simulink model "finalinversorPalacios"  (R2017a)
settings: Solver=ode3  StartTime=0.0  StopTime=10  MaxStep=1e-4  RelTol=1e-3
values from neighbouring files (symbols this model uses):
  Al = [0 -Uss/L; Uss/C -1/(R*C)]    [sistemacontrolado.m]    (also in sistemacontrolado.mat = [0  -0.441941738242; 441.941738242  -34.7222222222])
  Bl = [-X2ss/L; X1ss/C]    [sistemacontrolado.m]    (also in sistemacontrolado.mat = [-339.41125497 38.4])
  C = Ca1    (= 0.001)    [sistemacontrolado.m]    (also in sistemacontrolado.mat)
  C1 = 1.1e-6    (= 1.1e-06)    [sistemacontrolado.m]    (also in sistemacontrolado.mat)
  CI = x(end,1:2)    [sistemacontrolado.m]    (also in sistemacontrolado.mat = [0.0768083670357 339.401981032])
  Cl = [0 1]    [sistemacontrolado.m]    (also in sistemacontrolado.mat)
  I1 = 1.17    [sistemacontrolado.m]    (also in sistemacontrolado.mat)
  I2 = 3    [sistemacontrolado.m]    (also in sistemacontrolado.mat)
  Ki = k(1,3)    [sistemacontrolado.m]    (also in sistemacontrolado.mat = 8.5)
  Kp = k(1,1:2)    [sistemacontrolado.m]    (also in sistemacontrolado.mat = [-1.69344903458 -0.221299069674])
  L = 1    [sistemacontrolado.m]    (also in sistemacontrolado.mat)
  L1 = 4.5e-3    (= 0.0045)    [sistemacontrolado.m]    (also in sistemacontrolado.mat)
  La = 3e-3    (= 0.003)    [sistemacontrolado.m]    (also in sistemacontrolado.mat)
  R = Ra1    (= 28.8)    [sistemacontrolado.m]    (also in sistemacontrolado.mat)
  R1 = 1    [sistemacontrolado.m]    (also in sistemacontrolado.mat)
libraries: powerlib x56, fl_lib x5, nesl_utility x4, powerlib_extras x2, simulink x2, mpclib x1
settings Model: Creator=Administrador  LastModifiedBy=AndrewB
settings OptimizationCC: LifeSpan=inf
settings DebuggingCC: MaxConsecutiveZCsMsg=warning  SFExecutionAtInitializationDiag=none

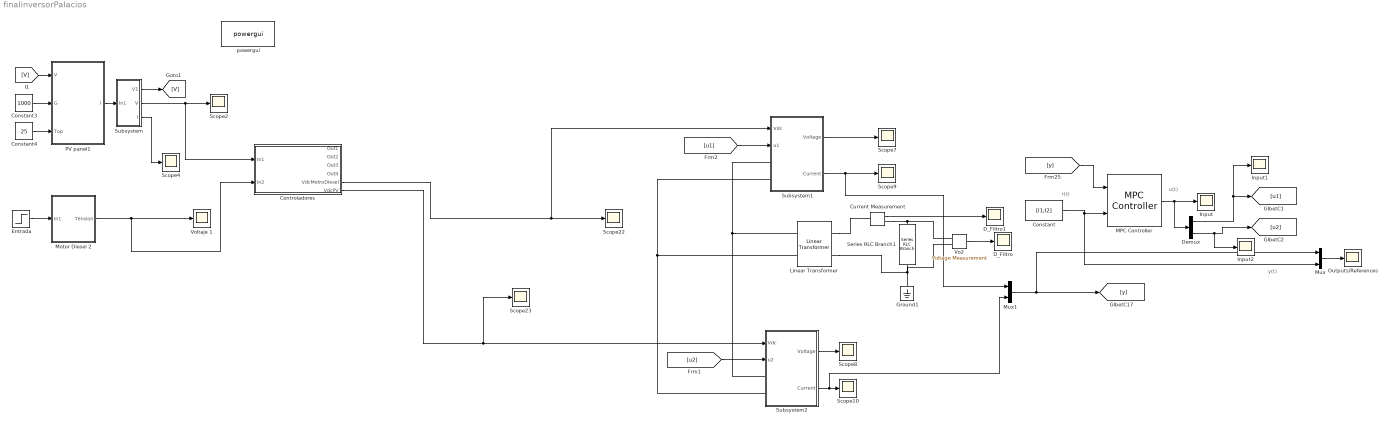
== system finalinversorPalacios ==
  note: u(t)
  note: y(t)
  note: r(t)
  Constant : Constant  Value=[I1;I2]
  Constant3 : Constant  Value=1000
  Constant4 : Constant  Value=25
  Controladores : Subsystem
  Current Measurement : powerlib/Measurements/Current Measurement  PhasorSimulation=off  OutputType=Complex  PSBequivalent=0
  D_Filtro : Scope
  D_Filtro1 : Scope
  Demux : Demux  Outputs=2
  Entrada : Step  Time=0  SampleTime=0
  Ground1 : powerlib/Elements/Ground  LConnTagsString=a
  Input : Scope
  Input1 : Scope
  Input2 : Scope
  Linear Transformer : powerlib/Elements/Linear Transformer  UNITS=SI  NominalPower=[ 1500 60 ]  winding1=[141.2 0 0.003]  winding2=[120 0.004 0.084225]  ThreeWindings=off  winding3=[3.15e+05 0.7938 0.084225]  RmLm=[1.0805e+06 2866]  Measurements=None  DataType=on
  MPC Controller : mpclib/MPC Controller  mpcobj=mpcobj  x0=[]  is_multiple=0  enable_value=0  return_u0=off  ref_from_ws=off  ref_signal_name=[]  ref_preview=on  md_from_ws=off  md_signal_name=[]  md_preview=on  from_project=off  project_file=MPCtask.mat  md_inport=off  mv_inport=off  cost_outport=off  return_sequence=off  return_qpstatus=off  return_state=off  state_inport=off  lims_inport=off  ywt_inport=off  is_designfromscratch=0  uwt_inport=off  duwt_inport=off  rhoeps_inport=off  uref_inport=off  n_ts=0.1  n_mv=2  n_md=0  n_ud=0  n_mo=2  n_uo=0  BlockDataType=double  SampleTimeInherited=off  switch_inport=off
  Motor Diesel 2 : Subsystem
  Mux : Mux  Inputs=2
  Mux1 : Mux  Inputs=2
  Outputs/References : Scope
  PV panel1 : Subsystem
      mask Display: image('panel.jpg')
  Scope{2,4,7..10,22..23} (8 alike) : Scope
  Series RLC Branch1 : powerlib/Elements/Series RLC Branch  LConnTagsString=__new0  RConnTagsString=__new0  BranchType=R  Resistance=R  Inductance=25e-3  SetiL0=off  InitialCurrent=0  Capacitance=5.30e-3  Setx0=off  InitialVoltage=0  Measurements=None
  Subsystem : Subsystem
  Subsystem1 : Subsystem
  Subsystem2 : Subsystem
  Vo2 : powerlib/Measurements/Voltage Measurement  PhasorSimulation=off  OutputType=Complex  PSBequivalent=0
  Voltaje 1 : Scope
  powergui : powerlib/powergui  SimulationMode=Discrete  SampleTime=1/60/10000  frequency=60  Iterations=50  frequencyindice=0  Pbase=100e6  ErrMax=1e-4  UnitsV=kV  UnitsW=MW  buscounter=0  FunctionMessages=off  echomessages=off  EnableUseOfTLC=off  CurrentSourceSwitches=off  DisableSnubberDevices=off  DisableRonSwitches=off  DisableVfSwitches=off  DisplayEquations=off  SolverType=Tustin/Backward Euler (TBE)  Interpol=off  ExternalGateDelay=off  methode=off  Ts=100  x0status=blocks  SPID=on  SwTol=0  HookPort=off  RestoreLinks=warning  ResistiveCurrentMeasurement=off  Frange=[0:2:500]  Ylog=off  Xlog=on  ShowGrid=off  save=off  variable=ZData  structure=sps1phPWM1_str  ZoomFFT=on  StartTime=0.1-2/60  cycles=2  DisplayStyle=1  fundamental=60  FreqAxis=off  MaxFrequency=5000  frequencyindicesteady=1  RmsSteady=1  display=off
  wires:
  [V] -> PV panel1/1(V)
  Subsystem/1(V1) -> [V]
  Constant4/1 -> PV panel1/3(Top)
  PV panel1/1(I) -> Subsystem/1(In1)
  Constant3/1 -> PV panel1/2(G)
  Subsystem/2(V) -> Controladores/1(In1), Scope2/1
  Subsystem/3(I) -> Scope4/1
  Entrada/1 -> Motor Diesel 2/1(In1)
  Motor Diesel 2/1(Tension) -> Controladores/2(In2), Voltaje 1/1
  Subsystem1/1(Voltage) -> Scope7/1
  Subsystem1/2(Current) -> Mux1/1, Scope9/1
  Vo2/1 -> D_Filtro/1
  Subsystem2/1(Voltage) -> Scope8/1
  Subsystem2/2(Current) -> Mux1/2, Scope10/1
  Current Measurement/1 -> D_Filtro1/1
  MPC Controller/1 -> Demux/1, Input/1
  Constant/1 -> Mux/2, MPC Controller/2
  Mux/1 -> Outputs/References/1
  [y] -> MPC Controller/1
  Mux1/1 -> Mux/1, [y]
  Demux/1 -> Input1/1, [u1]
  Demux/2 -> Input2/1, [u2]
  [u2] -> Subsystem2/2("u2 ")
  [u1] -> Subsystem1/2(u1)
  Controladores/5(VdcMotroDiesel) -> Subsystem1/1(Vdc), Scope22/1
  Controladores/6(VdcPV) -> Subsystem2/1(Vdc), Scope23/1
  connections:
  Subsystem1/LConn1 -- Subsystem2/LConn1 -- Linear Transformer/LConn1
  Subsystem1/LConn2 -- Subsystem2/LConn2 -- Linear Transformer/LConn2
  Vo2/LConn1 -- Current Measurement/RConn1 -- Series RLC Branch1/LConn1
  Ground1/LConn1 -- Linear Transformer/RConn2 -- Vo2/LConn2 -- Series RLC Branch1/RConn1
  Linear Transformer/RConn1 -- Current Measurement/LConn1

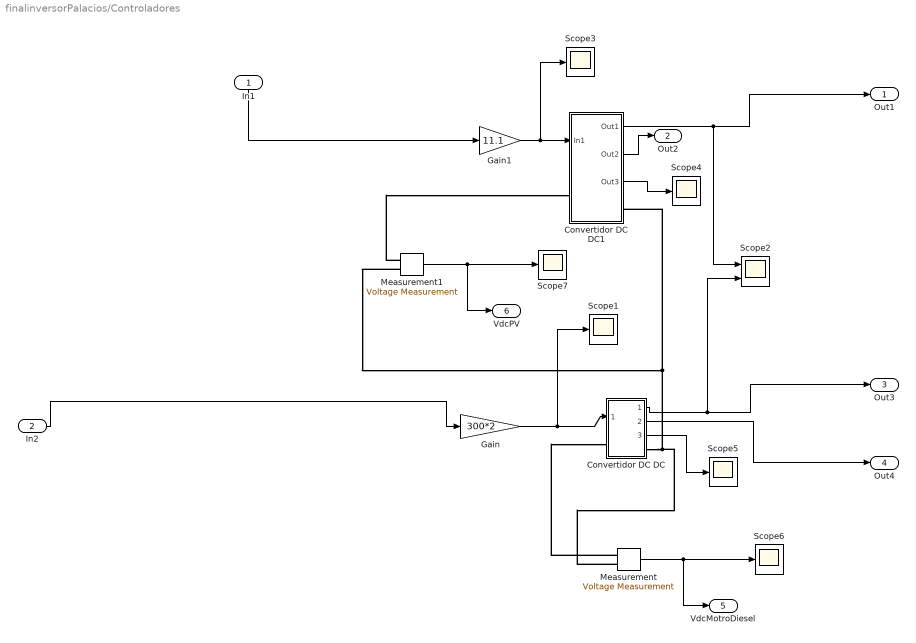
== system finalinversorPalacios/Controladores ==
  In1 : Inport
  In2 : Inport  Port=2
  " Measurement" : powerlib/Measurements/Voltage Measurement  PhasorSimulation=off  OutputType=Complex  PSBequivalent=0
  " Measurement1" : powerlib/Measurements/Voltage Measurement  PhasorSimulation=off  OutputType=Complex  PSBequivalent=0
  Convertidor DC DC : Subsystem
  Convertidor DC DC1 : Subsystem
  Gain : Gain  Gain=300*2
  Gain1 : Gain  Gain=11.1
  Scope{1,3..7} (6 alike) : Scope
  Scope2 : Scope  NumInputPorts=2
  Out1 : Outport
  Out2 : Outport  Port=2
  Out3 : Outport  Port=3
  Out4 : Outport  Port=4
  VdcMotroDiesel : Outport  Port=5
  VdcPV : Outport  Port=6
  wires:
  Gain/1 -> Scope1/1, Convertidor DC DC/1(In1)
  Convertidor DC DC/1(Out1) -> Scope2/2, Out3/1
  Convertidor DC DC1/1(Out1) -> Out1/1, Scope2/1
  Gain1/1 -> Scope3/1, Convertidor DC DC1/1(In1)
  Convertidor DC DC/2(Out2) -> Out4/1
  Convertidor DC DC1/2(Out2) -> Out2/1
  In1/1 -> Gain1/1
  In2/1 -> Gain/1
  Convertidor DC DC1/3(Out3) -> Scope4/1
  Convertidor DC DC/3(Out3) -> Scope5/1
  " Measurement"/1 -> VdcMotroDiesel/1, Scope6/1
  " Measurement1"/1 -> VdcPV/1, Scope7/1
  connections:
  Convertidor DC DC/RConn1 -- " Measurement"/LConn2 -- " Measurement1"/LConn2 -- Convertidor DC DC1/RConn1
  " Measurement"/LConn1 -- Convertidor DC DC/LConn1
  " Measurement1"/LConn1 -- Convertidor DC DC1/LConn1

== system finalinversorPalacios/Motor Diesel 2 ==
  In1 : Inport
  " Generador1" : Gain  Gain=1/2
  Actuador1 : TransferFcn  Denominator=[0.2 1]
  Control PI : TransferFcn  Numerator=[1 0.653]  Denominator=[1 0]
  Gain : Gain  Gain=3.87
  Inercia y fricción1 : TransferFcn  Denominator=[2.5 0.1]
  Scope1 : Scope
  Scope2 : Scope
  Scope3 : Scope
  Sistema de combustión1 : TransportDelay  DelayTime=0.1
  Sum : Sum  Inputs=|+-
  Tension : Outport
  wires:
  " Generador1"/1 -> Tension/1
  Actuador1/1 -> Sistema de combustión1/1, Scope2/1
  Gain/1 -> Control PI/1
  Sum/1 -> Gain/1
  Inercia y fricción1/1 -> Scope3/1, " Generador1"/1, Sum/2
  Control PI/1 -> Actuador1/1
  In1/1 -> Sum/1
  Sistema de combustión1/1 -> Inercia y fricción1/1, Scope1/1

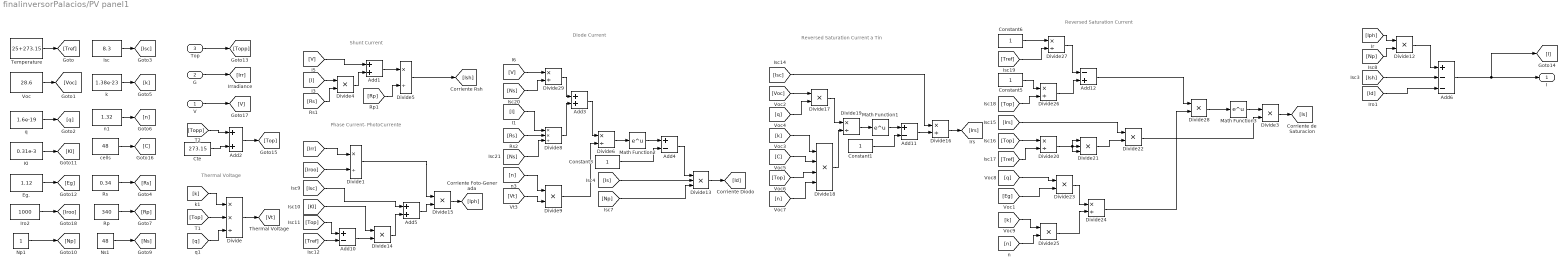
== system finalinversorPalacios/PV panel1 ==
  note: Thermal Voltage
  note: Shunt Current
  note: Phase Current- PhotoCurrente
  note: Diode Current
  note: Reversed Saturation Current a Tin
  note: Reversed Saturation Current
  V : Inport
  G : Inport  Port=2
  Top : Inport  Port=3
  Add{1..3,5} (4 alike) : Sum
  Add10 : Sum  Inputs=+-
  Add11 : Sum  Inputs=+-
  Add12 : Sum  Inputs=-+
  Add4 : Sum  Inputs=+-
  Add6 : Sum  Inputs=+--
  Constant{1,3,5..6} (4 alike) : Constant
  Cte : Constant  Value=273.15
  Divide : Product  Inputs=**/
  Divide{1,5..6,16,19..20,24,26..27,29} (10 alike) : Product  Inputs=*/
  Divide{3..4,9,12,14..15,17,22..23,25,28} (11 alike) : Product  Inputs=**
  Divide13 : Product  Inputs=***
  Divide18 : Product  Inputs=****
  Divide21 : Product  Inputs=***
  Divide8 : Product  Inputs=**/
  Eg. : Constant  Value=1.12
  Iro2 : Constant  Value=1000
  Isc : Constant  Value=8.3
  KI : Constant  Value=0.31e-3
  Math Function1 : Math  SaturateOnIntegerOverflow=on
  Math Function2 : Math  SaturateOnIntegerOverflow=on
  Math Function3 : Math  SaturateOnIntegerOverflow=on
  Np1 : Constant
  Ns1 : Constant  Value=48
  Rp : Constant  Value=340
  Rs : Constant  Value=0.34
  Temperature : Constant  Value=25+273.15
  Voc : Constant  Value=28.6
  cells : Constant  Value=48
  k : Constant  Value=1.38e-23
  n1 : Constant  Value=1.32
  q : Constant  Value=1.6e-19
  I : Outport
  wires:
  Temperature/1 -> [Tref]
  Voc/1 -> [Voc]
  q/1 -> [q]
  Isc/1 -> [Isc]
  k/1 -> [k]
  n1/1 -> [n]
  [k] -> Divide/1
  [Top] -> Divide/2
  [q] -> Divide/3
  Divide/1 -> [Vt]
  Divide3/1 -> [Is]
  [Ish] -> Add6/2
  Add6/1 -> I/1, [I]
  [I] -> Divide8/1
  [Rs] -> Divide8/2
  Divide8/1 -> Add3/2
  [n] -> Divide9/1
  [Vt] -> Divide9/2
  Divide9/1 -> Divide6/2
  Add3/1 -> Divide6/1
  Divide6/1 -> Math Function2/1
  Math Function2/1 -> Add4/1
  Add4/1 -> Divide13/1
  [Is] -> Divide13/2
  Divide13/1 -> [Id]
  Divide4/1 -> Add1/2
  Add1/1 -> Divide5/1
  [Rp] -> Divide5/2
  Divide5/1 -> [Ish]
  [Rs] -> Divide4/2
  [I] -> Divide4/1
  KI/1 -> [KI]
  Eg./1 -> [Eg]
  [V] -> Add1/1
  [Np] -> Divide13/3
  [Iph] -> Divide12/1
  [Np] -> Divide12/2
  Divide12/1 -> Add6/1
  [Isc] -> Add5/1
  [Top] -> Add10/1
  [Tref] -> Add10/2
  Add10/1 -> Divide14/2
  [KI] -> Divide14/1
  [Voc] -> Divide17/1
  [q] -> Divide17/2
  [k] -> Divide18/1
  [C] -> Divide18/2
  [Top] -> Divide18/3
  [n] -> Divide18/4
  Divide17/1 -> Divide19/1
  Divide18/1 -> Divide19/2
  Divide19/1 -> Math Function1/1
  Constant1/1 -> Add11/2
  Math Function1/1 -> Add11/1
  Add11/1 -> Divide16/2
  Divide16/1 -> [Irs]
  [Tref] -> Divide20/2
  [Top] -> Divide20/1
  Divide20/1 -> Divide21/2, Divide21/1, Divide21/3
  Divide21/1 -> Divide22/2
  [Irs] -> Divide22/1
  [q] -> Divide23/1
  Divide23/1 -> Divide24/1
  [k] -> Divide25/1
  [n] -> Divide25/2
  Divide25/1 -> Divide24/2
  Constant5/1 -> Divide26/1
  [Top] -> Divide26/2
  Constant6/1 -> Divide27/1
  [Tref] -> Divide27/2
  Divide27/1 -> Add12/1
  Divide26/1 -> Add12/2
  Add12/1 -> Divide28/1
  Divide24/1 -> Divide28/2
  Divide28/1 -> Math Function3/1
  Divide29/1 -> Add3/1
  [Ns] -> Divide29/2
  [V] -> Divide29/1
  [Ns] -> Divide8/3
  Divide14/1 -> Add5/2
  Add5/1 -> Divide15/2
  Divide15/1 -> [Iph]
  V/1 -> [V]
  G/1 -> [Irr]
  Top/1 -> [Topp]
  cells/1 -> [C]
  [Id] -> Add6/3
  Cte/1 -> Add2/2
  Add2/1 -> [Top]
  [Topp] -> Add2/1
  [Irr] -> Divide1/1
  [Iroo] -> Divide1/2
  Divide1/1 -> Divide15/1
  Iro2/1 -> [Iroo]
  Rs/1 -> [Rs]
  Rp/1 -> [Rp]
  Ns1/1 -> [Ns]
  Np1/1 -> [Np]
  Constant3/1 -> Add4/2
  [Isc] -> Divide16/1
  Math Function3/1 -> Divide3/1
  Divide22/1 -> Divide3/2
  [Eg] -> Divide23/2

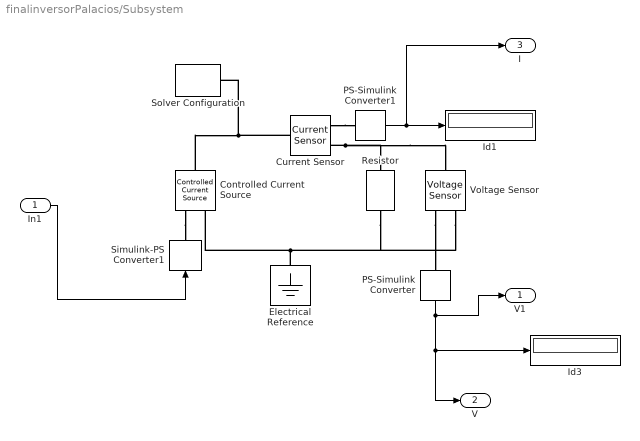
== system finalinversorPalacios/Subsystem ==
  In1 : Inport
  Controlled Current Source : fl_lib/Electrical/Electrical Sources/Controlled Current Source
  Current Sensor : fl_lib/Electrical/Electrical Sensors/Current Sensor
  Electrical Reference : fl_lib/Electrical/Electrical Elements/Electrical Reference
  Id1 : Display
  Id3 : Display
  PS-Simulink Converter : nesl_utility/PS-Simulink Converter  PhysicalDomain=network_engine_domain  SubClassName=ps_output  LeftPortType=input  RightPortType=output  PseudoPeriodic=off  Frequencies=[]  Unit=1  AffineConversion=off
  PS-Simulink Converter1 : nesl_utility/PS-Simulink Converter  PhysicalDomain=network_engine_domain  SubClassName=ps_output  LeftPortType=input  RightPortType=output  PseudoPeriodic=off  Frequencies=[]  Unit=1  AffineConversion=off
  Resistor : fl_lib/Electrical/Electrical Elements/Resistor  R=10.02 Ohm  i_specify=off  i_priority=High  i=0 A  i_nominal_specify=off  i_nominal_unit=A  i_nominal_value=1  v_specify=off  v_priority=High  v=0 V  v_nominal_specify=off  v_nominal_unit=V  v_nominal_value=1
  Simulink-PS Converter1 : nesl_utility/Simulink-PS Converter  PhysicalDomain=network_engine_domain  SubClassName=ps_input  LeftPortType=input  RightPortType=output  PseudoPeriodic=off  Frequencies=[]  NoiseDistribution=none  NoiseParameters=[]  Unit=1  AffineConversion=off  FilteringAndDerivatives=zero  SimscapeFilterOrder=1  InputFilterTimeConstant=.000001  UdotUserProvided=0
  Solver Configuration : nesl_utility/Solver Configuration  PhysicalDomain=network_engine_domain  SubClassName=solver  LeftPortType=input  RightPortType=generic  Accelerate=off  Tones=[]  Harmonics=[]  SimulateNoise=off  Profile=off  UseLocalSampling=off  EnableSwitchedLinearOptims=on  FrequencyDomain=off  UseCCode=off  RelTol=0.001  AbsTol=1e-06  MinStep=1e-09  ToWorkspace=off  RevertToSquareIcSolve=off  NumHomotopyIterations=100  PhasorMode=off  PhasorModeNumHarmonics=1  OverrideAbsTol=off  DoDC=on  ResidualTolerance=1e-8  UseLocalSolver=on  LocalSolverChoice=NE_BACKWARD_EULER_ADVANCER  LocalSolverSampleTime=.1  DoFixedCost=off  MaxNonlinIter=8  MaxModeIter=2  LinearAlgebra=Sparse  DelaysMemoryBudget=1024  AutomaticFiltering=on  FilteringTimeConstant=0.001
  Voltage Sensor : fl_lib/Electrical/Electrical Sensors/Voltage Sensor
  V1 : Outport
  V : Outport  Port=2
  I : Outport  Port=3
  wires:
  PS-Simulink Converter1/1 -> I/1, Id1/1
  PS-Simulink Converter/1 -> V1/1, V/1, Id3/1
  In1/1 -> Simulink-PS Converter1/1
  connections:
  Voltage Sensor/RConn1 -- PS-Simulink Converter/LConn1
  Current Sensor/RConn2 -- Voltage Sensor/LConn1 -- Resistor/LConn1
  Controlled Current Source/RConn1 -- Simulink-PS Converter1/RConn1
  Electrical Reference/LConn1 -- Voltage Sensor/RConn2 -- Resistor/RConn1 -- Controlled Current Source/RConn2
  Current Sensor/RConn1 -- PS-Simulink Converter1/LConn1
  Controlled Current Source/LConn1 -- Current Sensor/LConn1 -- Solver Configuration/RConn1

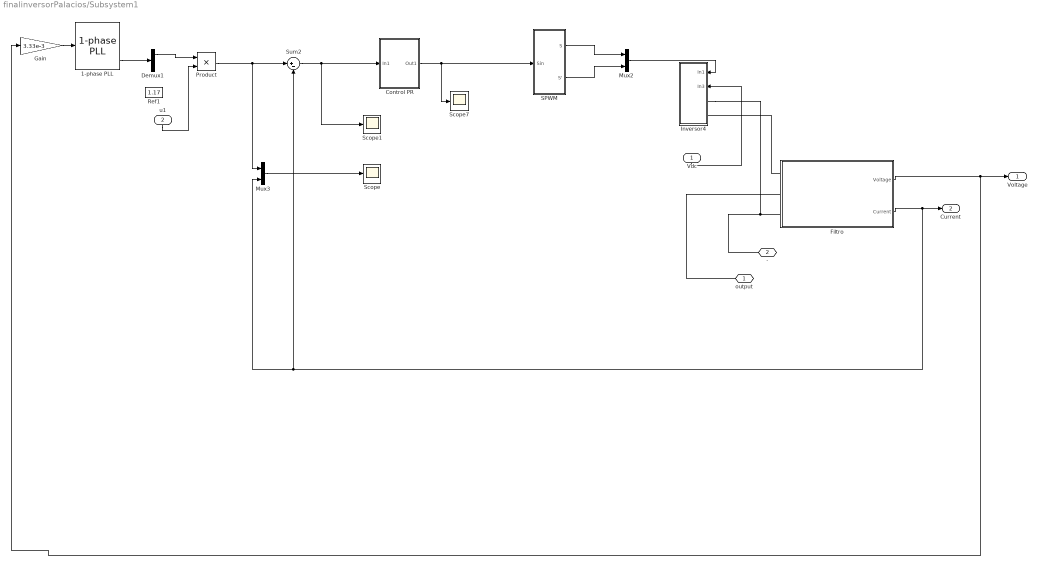
== system finalinversorPalacios/Subsystem1 ==
  Vdc : Inport
  u1 : Inport  Port=2
  1-phase PLL : powerlib_extras/Control  Blocks/1-phase PLL  Par_Init=[0 60]  ParK=[ 180 3200 1 ]  AGC=off
  Control PR : Subsystem
  Demux1 : Demux  Outputs=2
  Filtro : Subsystem
  Gain : Gain  Gain=3.33e-3
  Inversor4 : Subsystem
  Mux2 : Mux  Inputs=2
  Mux3 : Mux  Inputs=2
  Product : Product
  Ref1 : Constant  Value=1.17
  SPWM : Subsystem
  Scope : Scope
  Scope1 : Scope
  Scope7 : Scope
  Sum2 : Sum  Inputs=|+-
  output : PMIOPort  Port=1  Side=Left
  - : PMIOPort  Port=2  Side=Left
  Voltage : Outport
  Current : Outport  Port=2
  wires:
  Filtro/2(Current) -> Mux3/2, Sum2/2, Current/1
  Filtro/1(Voltage) -> Gain/1, Voltage/1
  1-phase PLL/3 -> Demux1/1
  Gain/1 -> 1-phase PLL/1
  Mux3/1 -> Scope/1
  Product/1 -> Mux3/1, Sum2/1
  Demux1/1 -> Product/1
  SPWM/1(S) -> Mux2/1
  SPWM/2(S') -> Mux2/2
  Mux2/1 -> Inversor4/1(In1)
  Vdc/1 -> Inversor4/2(In3)
  Control PR/1(Out1) -> Scope7/1, SPWM/1(Sin)
  Sum2/1 -> Scope1/1, Control PR/1(In1)
  u1/1 -> Product/2
  connections:
  output/RConn1 -- Filtro/LConn2
  -/RConn1 -- Inversor4/LConn1 -- Filtro/LConn3
  Filtro/LConn1 -- Inversor4/LConn2

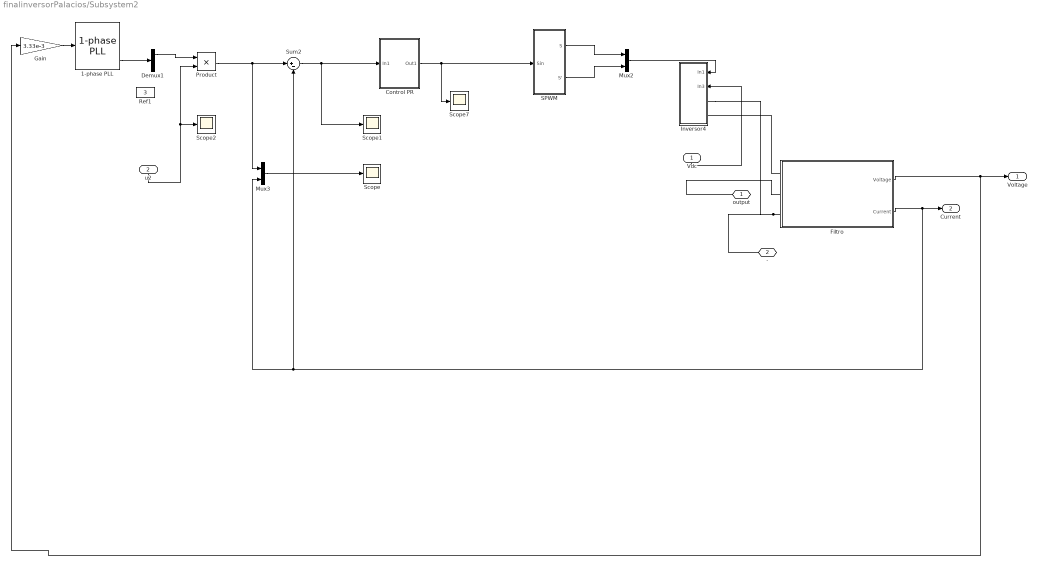
== system finalinversorPalacios/Subsystem2 ==
  Vdc : Inport
  "u2 " : Inport  Port=2
  1-phase PLL : powerlib_extras/Control  Blocks/1-phase PLL  Par_Init=[0 60]  ParK=[ 180 3200 1 ]  AGC=off
  Control PR : Subsystem
  Demux1 : Demux  Outputs=2
  Filtro : Subsystem
  Gain : Gain  Gain=3.33e-3
  Inversor4 : Subsystem
  Mux2 : Mux  Inputs=2
  Mux3 : Mux  Inputs=2
  Product : Product
  Ref1 : Constant  Value=3
  SPWM : Subsystem
  Scope{,1..2,7} (4 alike) : Scope
  Sum2 : Sum  Inputs=|+-
  output : PMIOPort  Port=1  Side=Left
  - : PMIOPort  Port=2  Side=Left
  Voltage : Outport
  Current : Outport  Port=2
  wires:
  Filtro/2(Current) -> Mux3/2, Sum2/2, Current/1
  Filtro/1(Voltage) -> Gain/1, Voltage/1
  1-phase PLL/3 -> Demux1/1
  Gain/1 -> 1-phase PLL/1
  Mux3/1 -> Scope/1
  Product/1 -> Mux3/1, Sum2/1
  Demux1/1 -> Product/1
  SPWM/1(S) -> Mux2/1
  SPWM/2(S') -> Mux2/2
  Mux2/1 -> Inversor4/1(In1)
  Vdc/1 -> Inversor4/2(In3)
  Control PR/1(Out1) -> Scope7/1, SPWM/1(Sin)
  Sum2/1 -> Scope1/1, Control PR/1(In1)
  "u2 "/1 -> Scope2/1, Product/2
  connections:
  output/RConn1 -- Filtro/LConn2
  Filtro/LConn3 -- -/RConn1 -- Inversor4/LConn1
  Filtro/LConn1 -- Inversor4/LConn2

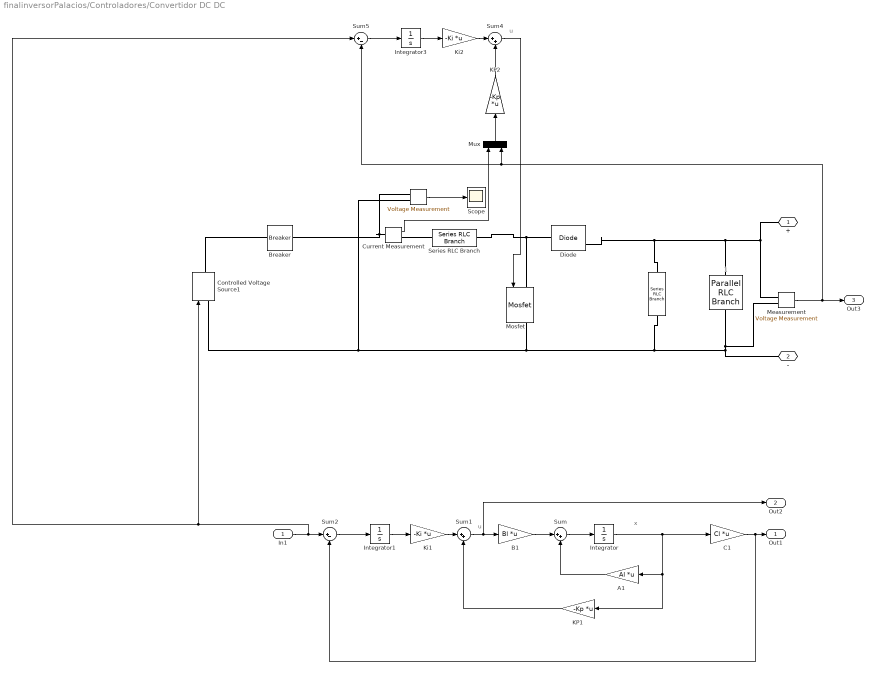
== system finalinversorPalacios/Controladores/Convertidor DC DC ==
  note: x
  note: u
  note: u
  In1 : Inport
  "  " : powerlib/Measurements/Voltage Measurement  PhasorSimulation=off  OutputType=Complex  PSBequivalent=0
  "    " : powerlib/Elements/Series RLC Branch  LConnTagsString=__new0  RConnTagsString=__new0  BranchType=C  Resistance=0  Inductance=69e-3  SetiL0=off  InitialCurrent=0  Capacitance=C  Setx0=off  InitialVoltage=0  Measurements=None
  "  1" : powerlib/Elements/Parallel RLC Branch  LConnTagsString=a  RConnTagsString=__new0  BranchType=R  Resistance=R  Inductance=1e-3  SetiL0=off  InitialCurrent=0  Capacitance=1e-6  Setx0=off  InitialVoltage=0  Measurements=None
  " Measurement" : powerlib/Measurements/Voltage Measurement  PhasorSimulation=off  OutputType=Complex  PSBequivalent=0
  A1 : Gain  Gain=Al  Multiplication=Matrix(K*u)
  B1 : Gain  Gain=Bl  Multiplication=Matrix(K*u)
  Breaker : powerlib/Elements/Breaker  InitialState=0  SwitchingTimes=[0 0.001]  External=off  BreakerResistance=0.01  SnubberResistance=1e6  SnubberCapacitance=inf  Measurements=None  MoreParameters=on  NoBreakLoop=off
      settings: SourceProductName=Simscape Power Systems
  C1 : Gain  Gain=Cl  Multiplication=Matrix(K*u)
  Controlled Voltage Source1 : powerlib/Electrical Sources/Controlled Voltage Source  Initialize=on  Source_Type=DC  Amplitude=0  Phase=0  Frequency=0  Measurements=None
  Current Measurement : powerlib/Measurements/Current Measurement  PhasorSimulation=off  OutputType=Complex  PSBequivalent=0
  Diode : powerlib/Power Electronics/Diode  Ron=0.001  Lon=0  Vf=0.8  IC=0  UseSnubber=off  Rs=500  Cs=250e-9  Measurements=on
  Integrator : Integrator  InitialCondition=CI
  Integrator1 : Integrator
  Integrator3 : Integrator
  KP1 : Gain  Gain=-Kp  Multiplication=Matrix(K*u)
  KP2 : Gain  Gain=-Kp  Multiplication=Matrix(K*u)
  Ki1 : Gain  Gain=-Ki  Multiplication=Matrix(K*u)
  Ki2 : Gain  Gain=-Ki  Multiplication=Matrix(K*u)
  Mosfet : powerlib/Power Electronics/Mosfet  Ron=0.1  Lon=0  Rd=0.01  Vfd=0  IC=0  Rs=1e5  Cs=inf  Measurements=on
  Mux : Mux  Inputs=2
  Scope : Scope
  Series RLC Branch : powerlib/Elements/Series RLC Branch  LConnTagsString=__new0  RConnTagsString=__new0  BranchType=L  Resistance=0  Inductance=L  SetiL0=off  InitialCurrent=0  Capacitance=1e-6  Setx0=off  InitialVoltage=0  Measurements=None
  Sum : Sum  Inputs=|++
  Sum1 : Sum  Inputs=|++
  Sum2 : Sum  Inputs=|+-
  Sum4 : Sum  Inputs=|++
  Sum5 : Sum  Inputs=|+-
  + : PMIOPort  Port=1  Side=Left
  - : PMIOPort  Port=2  Side=Right
  Out1 : Outport
  Out2 : Outport  Port=2
  Out3 : Outport  Port=3
  wires:
  Integrator1/1 -> Ki1/1
  B1/1 -> Sum/1
  Integrator/1 -> C1/1, KP1/1, A1/1
  Sum2/1 -> Integrator1/1
  Ki1/1 -> Sum1/1
  A1/1 -> Sum/2
  Sum/1 -> Integrator/1
  KP1/1 -> Sum1/2
  C1/1 -> Sum2/2, Out1/1
  Sum1/1 -> Out2/1, B1/1
  " Measurement"/1 -> Sum5/2, Mux/2, Out3/1
  In1/1 -> Sum5/1, Controlled Voltage Source1/1, Sum2/1
  "  "/1 -> Scope/1
  Mux/1 -> KP2/1
  Sum5/1 -> Integrator3/1
  Integrator3/1 -> Ki2/1
  Ki2/1 -> Sum4/1
  KP2/1 -> Sum4/2
  Sum4/1 -> Mosfet/1
  Current Measurement/1 -> Mux/1
  connections:
  Mosfet/RConn1 -- Controlled Voltage Source1/LConn1 -- "  "/LConn2 -- "    "/RConn1 -- -/RConn1 -- " Measurement"/LConn2 -- "  1"/RConn1
  "  1"/LConn1 -- +/RConn1 -- " Measurement"/LConn1 -- "    "/LConn1 -- Diode/RConn1
  Controlled Voltage Source1/RConn1 -- Breaker/LConn1
  Diode/LConn1 -- Series RLC Branch/RConn1 -- Mosfet/LConn1
  Current Measurement/RConn1 -- Series RLC Branch/LConn1
  Breaker/RConn1 -- Current Measurement/LConn1 -- "  "/LConn1

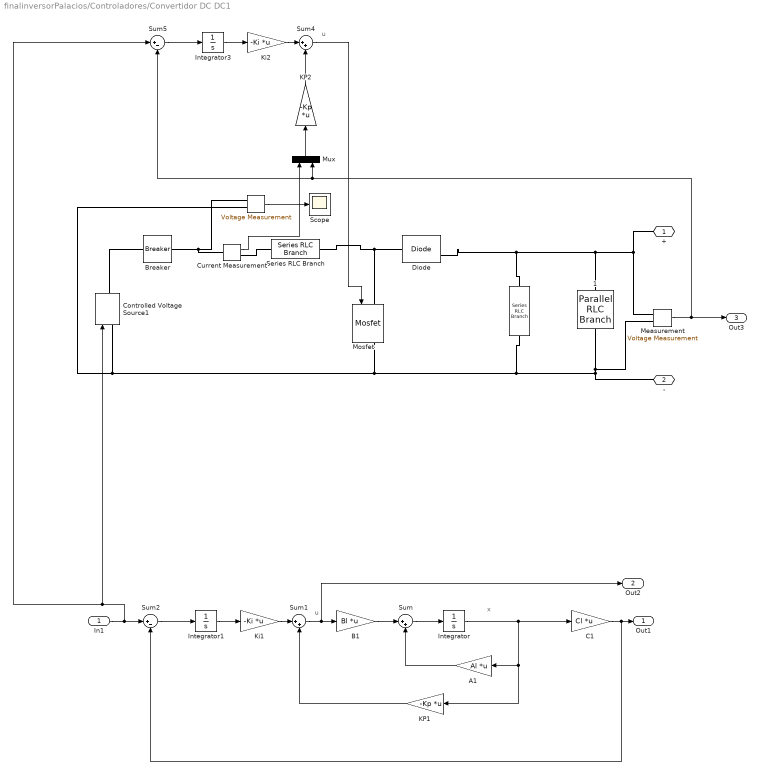
== system finalinversorPalacios/Controladores/Convertidor DC DC1 ==
  note: x
  note: u
  note: u
  In1 : Inport
  "  " : powerlib/Measurements/Voltage Measurement  PhasorSimulation=off  OutputType=Complex  PSBequivalent=0
  "    " : powerlib/Elements/Series RLC Branch  LConnTagsString=__new0  RConnTagsString=__new0  BranchType=C  Resistance=0  Inductance=69e-3  SetiL0=off  InitialCurrent=0  Capacitance=C  Setx0=off  InitialVoltage=0  Measurements=None
  "  1" : powerlib/Elements/Parallel RLC Branch  LConnTagsString=a  RConnTagsString=__new0  BranchType=R  Resistance=R  Inductance=1e-3  SetiL0=off  InitialCurrent=0  Capacitance=1e-6  Setx0=off  InitialVoltage=0  Measurements=None
  " Measurement" : powerlib/Measurements/Voltage Measurement  PhasorSimulation=off  OutputType=Complex  PSBequivalent=0
  A1 : Gain  Gain=Al  Multiplication=Matrix(K*u)
  B1 : Gain  Gain=Bl  Multiplication=Matrix(K*u)
  Breaker : powerlib/Elements/Breaker  InitialState=0  SwitchingTimes=[0 0.001]  External=off  BreakerResistance=0.01  SnubberResistance=1e6  SnubberCapacitance=inf  Measurements=None  MoreParameters=on  NoBreakLoop=off
      settings: SourceProductName=Simscape Power Systems
  C1 : Gain  Gain=Cl  Multiplication=Matrix(K*u)
  Controlled Voltage Source1 : powerlib/Electrical Sources/Controlled Voltage Source  Initialize=on  Source_Type=DC  Amplitude=0  Phase=0  Frequency=0  Measurements=None
  Current Measurement : powerlib/Measurements/Current Measurement  PhasorSimulation=off  OutputType=Complex  PSBequivalent=0
  Diode : powerlib/Power Electronics/Diode  Ron=0.001  Lon=0  Vf=0.8  IC=0  UseSnubber=off  Rs=500  Cs=250e-9  Measurements=on
  Integrator : Integrator  InitialCondition=CI
  Integrator1 : Integrator
  Integrator3 : Integrator
  KP1 : Gain  Gain=-Kp  Multiplication=Matrix(K*u)
  KP2 : Gain  Gain=-Kp  Multiplication=Matrix(K*u)
  Ki1 : Gain  Gain=-Ki  Multiplication=Matrix(K*u)
  Ki2 : Gain  Gain=-Ki  Multiplication=Matrix(K*u)
  Mosfet : powerlib/Power Electronics/Mosfet  Ron=0.1  Lon=0  Rd=0.01  Vfd=0  IC=0  Rs=1e5  Cs=inf  Measurements=on
  Mux : Mux  Inputs=2
  Scope : Scope
  Series RLC Branch : powerlib/Elements/Series RLC Branch  LConnTagsString=__new0  RConnTagsString=__new0  BranchType=L  Resistance=0  Inductance=L  SetiL0=off  InitialCurrent=0  Capacitance=1e-6  Setx0=off  InitialVoltage=0  Measurements=None
  Sum : Sum  Inputs=|++
  Sum1 : Sum  Inputs=|++
  Sum2 : Sum  Inputs=|+-
  Sum4 : Sum  Inputs=|++
  Sum5 : Sum  Inputs=|+-
  + : PMIOPort  Port=1  Side=Left
  - : PMIOPort  Port=2  Side=Right
  Out1 : Outport
  Out2 : Outport  Port=2
  Out3 : Outport  Port=3
  wires:
  Integrator1/1 -> Ki1/1
  B1/1 -> Sum/1
  Integrator/1 -> C1/1, KP1/1, A1/1
  Sum2/1 -> Integrator1/1
  Ki1/1 -> Sum1/1
  A1/1 -> Sum/2
  Sum/1 -> Integrator/1
  KP1/1 -> Sum1/2
  C1/1 -> Sum2/2, Out1/1
  Sum1/1 -> Out2/1, B1/1
  In1/1 -> Sum5/1, Controlled Voltage Source1/1, Sum2/1
  "  "/1 -> Scope/1
  KP2/1 -> Sum4/2
  Integrator3/1 -> Ki2/1
  Sum5/1 -> Integrator3/1
  Ki2/1 -> Sum4/1
  Sum4/1 -> Mosfet/1
  Mux/1 -> KP2/1
  Current Measurement/1 -> Mux/1
  " Measurement"/1 -> Sum5/2, Mux/2, Out3/1
  connections:
  "  1"/RConn1 -- " Measurement"/LConn2 -- -/RConn1 -- "    "/RConn1 -- Mosfet/RConn1 -- Controlled Voltage Source1/LConn1 -- "  "/LConn2
  Diode/RConn1 -- "    "/LConn1 -- "  1"/LConn1 -- +/RConn1 -- " Measurement"/LConn1
  "  "/LConn1 -- Breaker/RConn1 -- Current Measurement/LConn1
  Diode/LConn1 -- Series RLC Branch/RConn1 -- Mosfet/LConn1
  Current Measurement/RConn1 -- Series RLC Branch/LConn1
  Controlled Voltage Source1/RConn1 -- Breaker/LConn1

== system finalinversorPalacios/Subsystem1/Control PR ==
  In1 : Inport
  Transfer Fcn3 : TransferFcn  Numerator=[700 0]  Denominator=[1 37.5 (2*pi*60)^2]
  Out1 : Outport
  wires:
  In1/1 -> Transfer Fcn3/1
  Transfer Fcn3/1 -> Out1/1

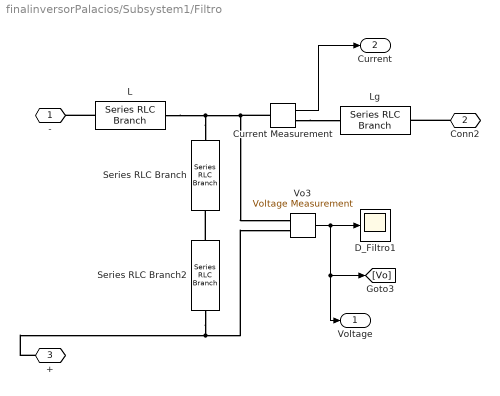
== system finalinversorPalacios/Subsystem1/Filtro ==
  Current Measurement : powerlib/Measurements/Current Measurement  PhasorSimulation=off  OutputType=Complex  PSBequivalent=0
  D_Filtro1 : Scope
  L : powerlib/Elements/Series RLC Branch  LConnTagsString=__new0  RConnTagsString=__new0  BranchType=RL  Resistance=0.01  Inductance=La  SetiL0=off  InitialCurrent=0  Capacitance=1e-6  Setx0=off  InitialVoltage=0  Measurements=None
  Lg : powerlib/Elements/Series RLC Branch  LConnTagsString=__new0  RConnTagsString=__new0  BranchType=RL  Resistance=R1  Inductance=L1  SetiL0=off  InitialCurrent=0  Capacitance=1e-6  Setx0=off  InitialVoltage=0  Measurements=None
  Series RLC Branch : powerlib/Elements/Series RLC Branch  LConnTagsString=__new0  RConnTagsString=__new0  BranchType=C  Resistance=10  Inductance=25e-3  SetiL0=off  InitialCurrent=0  Capacitance=C1  Setx0=on  InitialVoltage=0  Measurements=None
  Series RLC Branch2 : powerlib/Elements/Series RLC Branch  LConnTagsString=__new0  RConnTagsString=__new0  BranchType=R  Resistance=0.1  Inductance=25e-3  SetiL0=off  InitialCurrent=0  Capacitance=5.30e-3  Setx0=off  InitialVoltage=0  Measurements=None
  Vo3 : powerlib/Measurements/Voltage Measurement  PhasorSimulation=off  OutputType=Complex  PSBequivalent=0
  - : PMIOPort  Port=1  Side=Left
  Conn2 : PMIOPort  Port=2  Side=Left
  + : PMIOPort  Port=3  Side=Left
  Voltage : Outport
  Current : Outport  Port=2
  wires:
  Vo3/1 -> D_Filtro1/1, Voltage/1, [Vo]
  Current Measurement/1 -> Current/1
  connections:
  L/LConn1 -- -/RConn1
  Series RLC Branch/LConn1 -- Current Measurement/LConn1 -- Vo3/LConn1 -- L/RConn1
  Series RLC Branch2/LConn1 -- Series RLC Branch/RConn1
  Current Measurement/RConn1 -- Lg/LConn1
  Series RLC Branch2/RConn1 -- +/RConn1 -- Vo3/LConn2
  Conn2/RConn1 -- Lg/RConn1

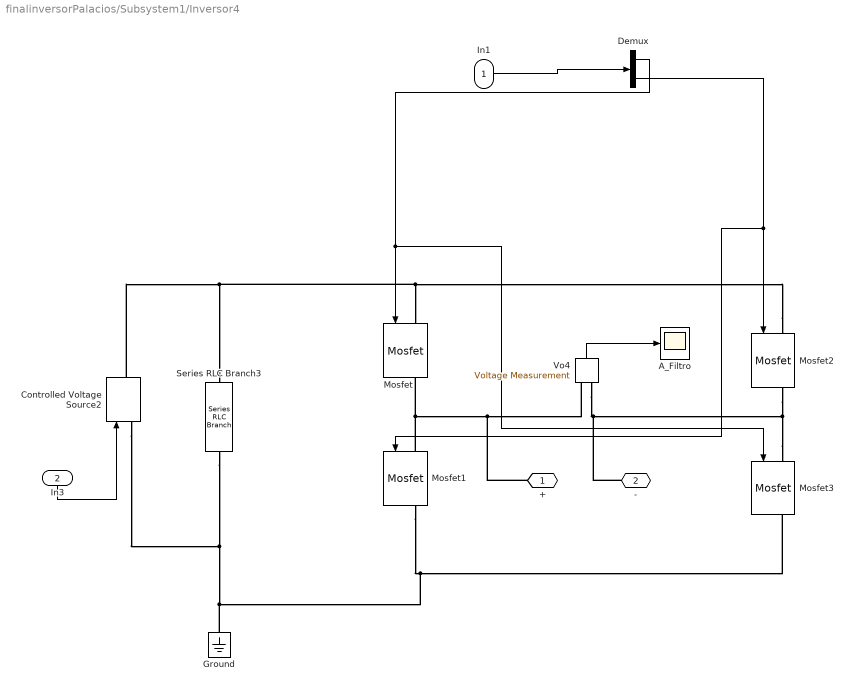
== system finalinversorPalacios/Subsystem1/Inversor4 ==
  In1 : Inport
  In3 : Inport  Port=2
  A_Filtro : Scope
  Controlled Voltage Source2 : powerlib/Electrical Sources/Controlled Voltage Source  Initialize=on  Source_Type=DC  Amplitude=0  Phase=0  Frequency=0  Measurements=None
  Demux : Demux  Outputs=2
  Ground : powerlib/Elements/Ground  LConnTagsString=a
  Mosfet{,1..3} (4 alike) : powerlib/Power Electronics/Mosfet  Ron=0.1  Lon=0  Rd=0.01  Vfd=0  IC=0  Rs=1e5  Cs=inf  Measurements=on
  Series RLC Branch3 : powerlib/Elements/Series RLC Branch  LConnTagsString=__new0  RConnTagsString=__new0  BranchType=RC  Resistance=1  Inductance=25e-3  SetiL0=off  InitialCurrent=0  Capacitance=2.2e-3  Setx0=off  InitialVoltage=0  Measurements=None
  Vo4 : powerlib/Measurements/Voltage Measurement  PhasorSimulation=off  OutputType=Complex  PSBequivalent=0
  + : PMIOPort  Port=1  Side=Left
  - : PMIOPort  Port=2  Side=Left
  wires:
  Vo4/1 -> A_Filtro/1
  Demux/1 -> Mosfet3/1, Mosfet/1
  Demux/2 -> Mosfet1/1, Mosfet2/1
  In3/1 -> Controlled Voltage Source2/1
  In1/1 -> Demux/1
  connections:
  Mosfet3/LConn1 -- -/RConn1 -- Vo4/LConn2 -- Mosfet2/RConn1
  Mosfet2/LConn1 -- Mosfet/LConn1 -- Controlled Voltage Source2/RConn1 -- Series RLC Branch3/LConn1
  Mosfet/RConn1 -- Mosfet1/LConn1 -- Vo4/LConn1 -- +/RConn1
  Mosfet1/RConn1 -- Series RLC Branch3/RConn1 -- Controlled Voltage Source2/LConn1 -- Ground/LConn1 -- Mosfet3/RConn1

== system finalinversorPalacios/Subsystem1/SPWM ==
  Sin : Inport
  10V~5KHz : simulink/Sources/Repeating Sequence  rep_seq_t=[0 0.0001 0.0002]  rep_seq_y=[-10.5 10.5 -10.5]
  Gain : Gain  Gain=10
  Gain1 : Gain  Gain=10
  Logical Operator : Logic  Operator=NOT  AllPortsSameDT=off  OutDataTypeStr=boolean
  Mux : Mux  Inputs=2
  Relational Operator : RelationalOperator  OutDataTypeStr=boolean  RndMeth=Nearest
  Scope1 : Scope
  Scope2 : Scope
  Scope4 : Scope
  S : Outport
  S' : Outport  Port=2
  wires:
  10V~5KHz/1 -> Relational Operator/1, Mux/1, Scope2/1
  Relational Operator/1 -> Gain/1, Logical Operator/1
  Logical Operator/1 -> Gain1/1
  Gain/1 -> S/1
  Gain1/1 -> S'/1
  Mux/1 -> Scope1/1
  Sin/1 -> Relational Operator/2, Mux/2
  ? -> Scope4/1

== system finalinversorPalacios/Subsystem2/Control PR ==
  In1 : Inport
  Transfer Fcn3 : TransferFcn  Numerator=[700 0]  Denominator=[1 37.5 (2*pi*60)^2]
  Out1 : Outport
  wires:
  In1/1 -> Transfer Fcn3/1
  Transfer Fcn3/1 -> Out1/1

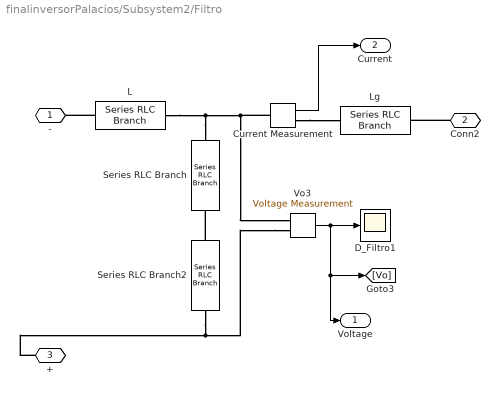
== system finalinversorPalacios/Subsystem2/Filtro ==
  Current Measurement : powerlib/Measurements/Current Measurement  PhasorSimulation=off  OutputType=Complex  PSBequivalent=0
  D_Filtro1 : Scope
  L : powerlib/Elements/Series RLC Branch  LConnTagsString=__new0  RConnTagsString=__new0  BranchType=RL  Resistance=0.01  Inductance=La  SetiL0=off  InitialCurrent=0  Capacitance=1e-6  Setx0=off  InitialVoltage=0  Measurements=None
  Lg : powerlib/Elements/Series RLC Branch  LConnTagsString=__new0  RConnTagsString=__new0  BranchType=RL  Resistance=R1  Inductance=L1  SetiL0=off  InitialCurrent=0  Capacitance=1e-6  Setx0=off  InitialVoltage=0  Measurements=None
  Series RLC Branch : powerlib/Elements/Series RLC Branch  LConnTagsString=__new0  RConnTagsString=__new0  BranchType=C  Resistance=10  Inductance=25e-3  SetiL0=off  InitialCurrent=0  Capacitance=C1  Setx0=on  InitialVoltage=0  Measurements=None
  Series RLC Branch2 : powerlib/Elements/Series RLC Branch  LConnTagsString=__new0  RConnTagsString=__new0  BranchType=R  Resistance=0.1  Inductance=25e-3  SetiL0=off  InitialCurrent=0  Capacitance=5.30e-3  Setx0=off  InitialVoltage=0  Measurements=None
  Vo3 : powerlib/Measurements/Voltage Measurement  PhasorSimulation=off  OutputType=Complex  PSBequivalent=0
  - : PMIOPort  Port=1  Side=Left
  Conn2 : PMIOPort  Port=2  Side=Left
  + : PMIOPort  Port=3  Side=Left
  Voltage : Outport
  Current : Outport  Port=2
  wires:
  Vo3/1 -> D_Filtro1/1, Voltage/1, [Vo]
  Current Measurement/1 -> Current/1
  connections:
  L/LConn1 -- -/RConn1
  Series RLC Branch/LConn1 -- Current Measurement/LConn1 -- Vo3/LConn1 -- L/RConn1
  Series RLC Branch2/LConn1 -- Series RLC Branch/RConn1
  Current Measurement/RConn1 -- Lg/LConn1
  Vo3/LConn2 -- Series RLC Branch2/RConn1 -- +/RConn1
  Conn2/RConn1 -- Lg/RConn1

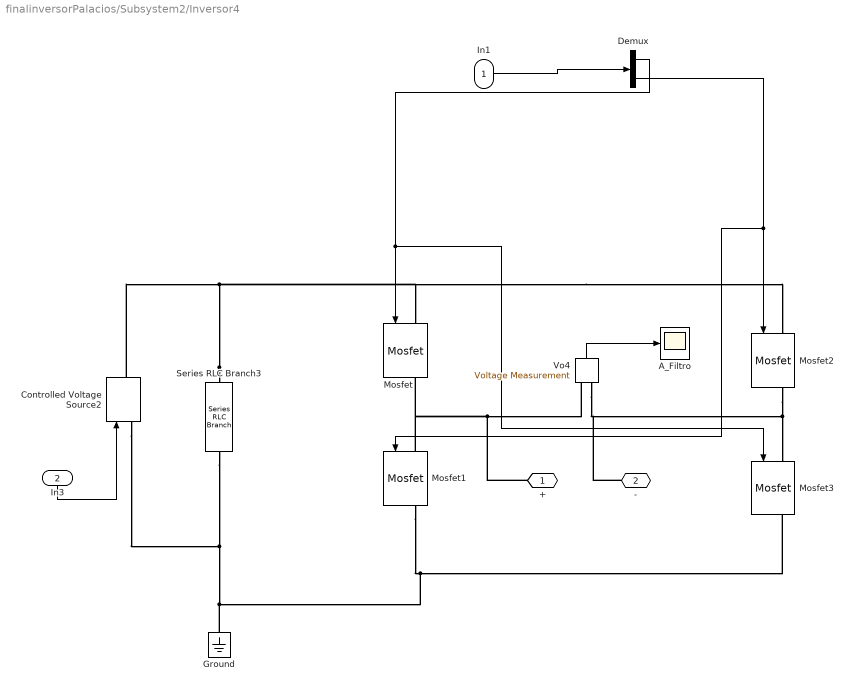
== system finalinversorPalacios/Subsystem2/Inversor4 ==
  In1 : Inport
  In3 : Inport  Port=2
  A_Filtro : Scope
  Controlled Voltage Source2 : powerlib/Electrical Sources/Controlled Voltage Source  Initialize=on  Source_Type=DC  Amplitude=0  Phase=0  Frequency=0  Measurements=None
  Demux : Demux  Outputs=2
  Ground : powerlib/Elements/Ground  LConnTagsString=a
  Mosfet{,1..3} (4 alike) : powerlib/Power Electronics/Mosfet  Ron=0.1  Lon=0  Rd=0.01  Vfd=0  IC=0  Rs=1e5  Cs=inf  Measurements=on
  Series RLC Branch3 : powerlib/Elements/Series RLC Branch  LConnTagsString=__new0  RConnTagsString=__new0  BranchType=RC  Resistance=1  Inductance=25e-3  SetiL0=off  InitialCurrent=0  Capacitance=2.2e-3  Setx0=off  InitialVoltage=0  Measurements=None
  Vo4 : powerlib/Measurements/Voltage Measurement  PhasorSimulation=off  OutputType=Complex  PSBequivalent=0
  + : PMIOPort  Port=1  Side=Left
  - : PMIOPort  Port=2  Side=Left
  wires:
  Vo4/1 -> A_Filtro/1
  Demux/1 -> Mosfet3/1, Mosfet/1
  Demux/2 -> Mosfet1/1, Mosfet2/1
  In3/1 -> Controlled Voltage Source2/1
  In1/1 -> Demux/1
  connections:
  Mosfet2/RConn1 -- Mosfet3/LConn1 -- Vo4/LConn2 -- -/RConn1
  Series RLC Branch3/LConn1 -- Mosfet/LConn1 -- Mosfet2/LConn1 -- Controlled Voltage Source2/RConn1
  +/RConn1 -- Mosfet1/LConn1 -- Mosfet/RConn1 -- Vo4/LConn1
  Series RLC Branch3/RConn1 -- Mosfet3/RConn1 -- Mosfet1/RConn1 -- Ground/LConn1 -- Controlled Voltage Source2/LConn1

== system finalinversorPalacios/Subsystem2/SPWM ==
  Sin : Inport
  10V~5KHz : simulink/Sources/Repeating Sequence  rep_seq_t=[0 0.0001 0.0002]  rep_seq_y=[-10.5 10.5 -10.5]
  Gain : Gain  Gain=10
  Gain1 : Gain  Gain=10
  Logical Operator : Logic  Operator=NOT  AllPortsSameDT=off  OutDataTypeStr=boolean
  Mux : Mux  Inputs=2
  Relational Operator : RelationalOperator  OutDataTypeStr=boolean  RndMeth=Nearest
  Scope1 : Scope
  Scope2 : Scope
  Scope4 : Scope
  S : Outport
  S' : Outport  Port=2
  wires:
  10V~5KHz/1 -> Relational Operator/1, Mux/1, Scope2/1
  Relational Operator/1 -> Gain/1, Logical Operator/1
  Logical Operator/1 -> Gain1/1
  Gain/1 -> S/1
  Gain1/1 -> S'/1
  Mux/1 -> Scope1/1
  Sin/1 -> Relational Operator/2, Mux/2
  ? -> Scope4/1
